simulink model "sim_model"  (R2023b)
settings: Solver=ode15s  StartTime=0.0  StopTime=T_sim  FixedStep=1e-4  RelTol=1e-6
undefined symbols (not defined in the file): A, B, Bw, C, D, Dw, K, Pi_yu, Qu, Qy, w_const, x0
settings Model: Creator=fjako  LastModifiedBy=fjako

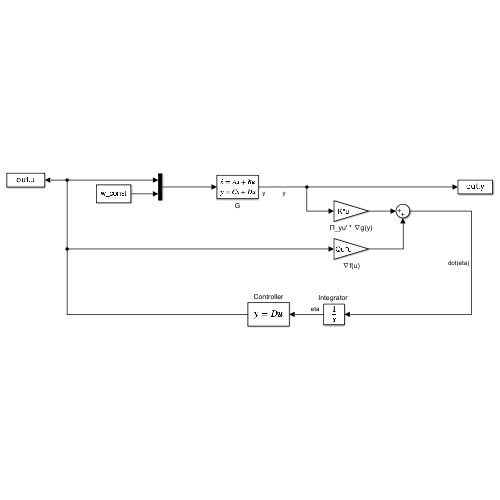
[thumbnail: Simulink's stored preview of the top-level diagram]
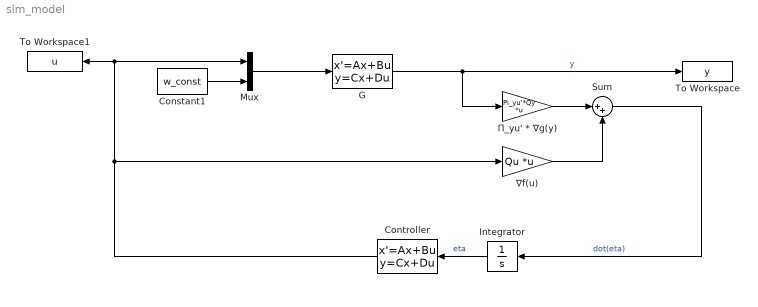
== system sim_model ==
  Constant1 : Constant  Value=w_const
  Controller : StateSpace  A=K.A  B=K.B  C=K.C  D=K.D  InitialCondition=0
  G : StateSpace  A=A  B=[B Bw]  C=C  D=[D Dw]  InitialCondition=x0
  "Integrator " : Integrator
  Mux : Mux  Inputs=2
  Sum : Sum  Inputs=|++
  To Workspace : ToWorkspace  VariableName=y  SaveFormat=Timeseries  SampleTime=-1
  To Workspace1 : ToWorkspace  VariableName=u  SaveFormat=Timeseries  SampleTime=-1
  Π_yu' * ∇g(y) : Gain  Gain=Pi_yu'*Qy  Multiplication=Matrix(K*u)
  ∇f(u) : Gain  Gain=Qu  Multiplication=Matrix(K*u)
  wires:
  Constant1/1 -> Mux/2
  Controller/1 -> Mux/1, To Workspace1/1, ∇f(u)/1
  Π_yu' * ∇g(y)/1 -> Sum/1
  ∇f(u)/1 -> Sum/2
  Sum/1 -> "Integrator "/1  "dot(eta)"
  G/1 -> Π_yu' * ∇g(y)/1, To Workspace/1  "y"
  Mux/1 -> G/1
  "Integrator "/1 -> Controller/1  "eta"
